simulink model "Control_test"  (R2014b)
settings: Solver=FixedStepDiscrete  StartTime=0.0  StopTime=Inf  FixedStep=0.001  RelTol=1e-3
PostLoadFcn:
  | , if any(exist('dsrtsu_mdlpostloadfcn', 'file') == [2, 3, 6]), try dsrtsu_mdlpostloadfcn('Execute', bdroot); catch fprintf('Error in PostLoadFcn (dsrtsu_mdlpostloadfcn) for model "%s":\n %s\n', bdroot, lasterr); end, end,
undefined symbols (not defined in the file or in its folder): dtLocal, slcm
libraries: rtican x163, simulink x14
(part 15 of 34)

== system Control_test/InputProcessing/RadarCanProcessing/ESR_Status5 ==
  Bus Creator : BusCreator  Inputs=8
  ESR_Status5 : rtican/RTICAN Receive (RX)   Reserved1=[]  Reserved2=[]  Reserved3=[]  Reserved4=[]  SfcnMessage=[]  Msg_Struct=[]  BoardTypeNo=[]  BoardNo=[]  ChannelNo=[]  Parameters=[]  DialogFcn=[]  UnitName=[]  Revision=[]  UnitValues=[]  DSProperties=struct('RTI',struct('Version',uint32(5),'BlockType',struct('isSLSource',uint8(1),'isSLSink',uint8(1),'isHWSource',uint8(0),'isHWSink',uint8(0),'isSetup',uint8(0),'isInline',uint8(1),'isNonInline',uint8(0),'isInterrupt',uint8(0),'isChannelwise',uint8(0)),'IOBoardType','RTICAN','UnitType','MESSAGE','Identifier','RX','DialogType','MSVC','BlockSet','RTICAN','SlaveProcessor','CAN'))  RTIBlockInterface=struct('OutputPortsWidth',int32([1 1 1 1 1 1 1 1]),'OutputPortsActive',[1 1 1 1 1 1 1 1],'OutputPortsName',{{'CAN_TX_SUPPLY_10V_A2D','CAN_TX_SUPPLY_3P3V_A2D','CAN_TX_SUPPLY_5VDX_A2D','CAN_TX_SUPPLY_5VA_A2D','CAN_TX_TEMP2_A2D','CAN_TX_TEMP1_A2D','CAN_TX_IGNP_A2D','CAN_TX_SWBATT_A2D'}},'OutputPortsDataType',{{'SS_DOUBLE','SS_DOUBLE','SS_DOUBLE','SS_DOUBLE','SS_DOUBLE','SS_DOUBLE','SS_DOUBLE','SS_DOUBLE'}},'OutputPortsLabel',{{'CAN_TX_SUPPLY_10V_A2D','CAN_TX_SUPPLY_3P3V_A2D','CAN_TX_SUPPLY_5VDX_A2D','CAN_TX_SUPPLY_5VA_A2D','CAN_TX_TEMP2_A2D','CAN_TX_TEMP1_A2D','CAN_TX_IGNP_A2D','CAN_TX_SWBATT_A2D'}},'OutputPortsLabelMode','ON','InputPortsWidth',int32(0),'InputPortsActive',0,'DialogFcn','rtican_message_interface_gui','BlockDisplay',{{'','center'}},'IconTransparency','on','ParameterTunableNames',{{}},'InitLevel',3,'BlockName',struct('Token',{{'ESR_Status5'}}),'SampleTime',{{-1}},'TriggerPort',{{'none'}},'EnablePort',{{'none'}})  RTIBlockParameters=struct('BoardTypeNo',{{1,'OFF',[]}},'BoardNo',{{2,'ON',[1 16]}},'ChannelNo',{{2,'ON',[1 2]}},'Parameters',{{struct('DataFileSupport',struct('DataFileSelectedMaster',1,'DataFileSelectedLocal',1,'DataFileName',['c:\users\mpc\dropbox\hyundai car setup\esr_dv3_64tgt.dbc|'],'DataFileDate',['26-Aug-2014 13:16:21'],'SelectedFile','..\..\dbcfiles\esr_dv3_64tgt.dbc','InterfaceFcn','rtican_dbc_file_parser'),'Options',struct('StatusSelected',0,'TimeSelected',0,'DeltaTimeSelected',0,'BytePortSelected',0,'MessageLengthSelected',0,'TriggerPort',struct('Selected',0,'TriggerType',0),'UserCoding',struct('Selected',0,'InterfaceFile','UserDecodingFile','FcnName','UserDecodeFcn','InportSelected',0,'InportWidth',1,'OutportSelected',0,'OutportWidth',1),'EnablePortSelected',0,'SignalOnPortnameSelected',1,'UseRXService',0),'Message',struct('MsgOnBlocknameSelected',1,'MsgName','ESR_Status5','MsgIdFormat',0,'MsgId',1508,'MsgLength',8,'NumSignals',8,'SampleTime',-1,'Signal',struct('SgnName',{'CAN_TX_SUPPLY_10V_A2D','CAN_TX_SUPPLY_3P3V_A2D','CAN_TX_SUPPLY_5VDX_A2D','CAN_TX_SUPPLY_5VA_A2D','CAN_TX_TEMP2_A2D','CAN_TX_TEMP1_A2D','CAN_TX_IGNP_A2D','CAN_TX_SWBATT_A2D'},'SgnStartBit',{0,8,16,24,32,40,48,56},'SgnLength',{8,8,8,8,8,8,8,8},'ByteLayout',{2,2,2,2,2,2,2,2},'Factor',{1,1,1,1,1,1,1,1},'Offset',{0,0,0,0,0,0,0,0},'SgnComment',{'','','','','','','',''},'SgnUnit',{'','','','','','','',''},'Min',{0,0,0,0,0,0,0,0},'Max',{0,0,0,0,0,0,0,0},'SgnType',{0,0,0,0,0,0,0,0},'SLDataType',{'SS_DOUBLE','SS_DOUBLE','SS_DOUBLE','SS_DOUBLE','SS_DOUBLE','SS_DOUBLE','SS_DOUBLE','SS_DOUBLE'},'DataType',{0,0,0,0,0,0,0,0},'ModeValue',{-1,-1,-1,-1,-1,-1,-1,-1}),'MsgIdNumFormat',0,'MsgComment',{{''}}),'Version',1.2,'general',struct('isFromLib',0)),'OFF',[]}},'GroupId',{{struct('Group',{{'RTICAN'}},'No',4,'Behavior',{{'NAMECHANGE'}},'BlockType',{{'SINK'}},'NameChangeFlag',0),'OFF',[]}},'SFcnRTICANMessage',{{struct('MsgType','RX','SFcnPortType','Scalar','MsgName','ESR_Status5','MsgIdFormat','STD','MsgId',1508,'MsgLength',8,'NumSignals',8,'SampleTime',-1,'Signal',struct('SgnName',{'CAN_TX_SUPPLY_10V_A2D','CAN_TX_SUPPLY_3P3V_A2D','CAN_TX_SUPPLY_5VDX_A2D','CAN_TX_SUPPLY_5VA_A2D','CAN_TX_TEMP2_A2D','CAN_TX_TEMP1_A2D','CAN_TX_IGNP_A2D','CAN_TX_SWBATT_A2D'},'SgnStartBit',{0,8,16,24,32,40,48,56},'SgnLength',{8,8,8,8,8,8,8,8},'ByteLayout',{['motorola back.'],['motorola back.'],['motorola back.'],['motorola back.'],['motorola back.'],['motorola back.'],['motorola back.'],['motorola back.']},'Factor',{1,1,1,1,1,1,1,1},'Offset',{0,0,0,0,0,0,0,0},'SgnType',{'standard','standard','standard','standard','standard','standard','standard','standard'},'SLDataType',{'SS_DOUBLE','SS_DOUBLE','SS_DOUBLE','SS_DOUBLE','SS_DOUBLE','SS_DOUBLE','SS_DOUBLE','SS_DOUBLE'},'DataType',{['unsigned int'],['unsigned int'],['unsigned int'],['unsigned int'],['unsigned int'],['unsigned int'],['unsigned int'],['unsigned int']},'ModeValue',{-1,-1,-1,-1,-1,-1,-1,-1}),'StatusSelected','no','TimeSelected','no','DeltaTimeSelected','no','BytePortSelected','no','MessageLengthSelected','no','TriggerPort',struct('Selected','no','TriggerType',0),'UserCoding',struct('Selected','no','InterfaceFile','UserDecodingFile','FcnName','UserDecodeFcn','InportSelected','no','InportWidth',1,'OutportSelected','no','OutportWidth',1),'EnablePortSelected','no','UseRXService','no','BoardType','DS1','BoardNo',2,'ControllerNo',2),'OFF',[]}},'TLCFileName',{{'rtican_rx_message','OFF',[]}})  RTISFcnParameters=struct('SFcnRTICANMessage','struct','TLCFileName','char')  RTIBlockParaDefault=struct('BoardTypeNo',4302,'BoardNo',1,'ChannelNo',1,'Parameters',struct('DataFileSupport',struct('DataFileSelectedMaster',0,'DataFileSelectedLocal',0,'DataFileName','','DataFileDate','','SelectedFile',['<no file selected>']),'Options',struct('StatusSelected',1,'TimeSelected',1,'DeltaTimeSelected',1,'BytePortSelected',0,'MessageLengthSelected',0,'TriggerPort',struct('Selected',0,'TriggerType','rising'),'UserCoding',struct('Selected',0,'InterfaceFile','UserDecodingFile','FcnName','UserDecodeFcn','InportSelected',0,'InportWidth',1,'OutportSelected',0,'OutportWidth',1),'EnablePortSelected',0,'SignalOnPortnameSelected',1,'UseRXService',0),'Message',struct('MsgOnBlocknameSelected',0,'MsgName',['RX Message'],'MsgIdFormat',0,'MsgId',100,'MsgLength',8,'NumSignals',1,'SampleTime',-1,'Signal',struct('SgnName',['RX signal'],'SgnStartBit',0,'SgnLength',8,'SgnType',0,'ModeValue',-1,'DataType',0,'SLDataType','SS_DOUBLE','ByteLayout',0,'Factor',1,'Offset',0,'Min',0,'Max',255,'SgnComment',{{}},'SgnUnit',''),'MsgIdNumFormat',0,'MsgComment',{{''}}),'Version',1.2,'general',struct('isFromLib',1)),'GroupId',struct('Group',{{'RTICAN'}},'No',1,'Behavior',{{'NAMECHANGE'}},'BlockType',{{'SINK'}},'NameChangeFlag',0),'SFcnRTICANMessage',struct('MsgType','RX','MsgName',['RX Message'],'MsgIdFormat','STD','MsgId',100,'MsgLength',8,'NumSignals',1,'SampleTime',-1,'Signal',struct('SgnName',['RX signal'],'SgnStartBit',0,'SgnLength',8,'SgnType','standard','ModeValue',-1,'DataType',['unsigned int'],'ByteLayout',['little endian'],'SLDataType','SS_DOUBLE','Factor',1,'Offset',0),'StatusSelected','yes','TimeSelected','yes','DeltaTimeSelected','yes','BytePortSelected','no','MessageLengthSelected','no','EnablePortSelected','no','UserCoding',struct('Selected','no','InterfaceFile','UserDecodingFile','FcnName','UserDecodeFcn','InportSelected','no','InportWidth',1,'OutportSelected','no','OutportWidth',1),'TriggerPort',struct('Selected','no','TriggerType','rising'),'UseRXService','no','BoardType','DS4302','BoardNo',1,'ControllerNo',1,'SFcnPortType','Scalar'),'TLCFileName','rtican_rx_message')
      settings: AttributesFormatString=Group Id: RTICAN4\n
  ESR_Status5_1 : Outport
  wires:
  Bus Creator/1 -> ESR_Status5_1/1  "ESR_Status5"
  ESR_Status5/1 -> Bus Creator/1  "CAN_TX_SUPPLY_10V_A2D"
  ESR_Status5/2 -> Bus Creator/2  "CAN_TX_SUPPLY_3P3V_A2D"
  ESR_Status5/3 -> Bus Creator/3  "CAN_TX_SUPPLY_5VDX_A2D"
  ESR_Status5/4 -> Bus Creator/4  "CAN_TX_SUPPLY_5VA_A2D"
  ESR_Status5/5 -> Bus Creator/5  "CAN_TX_TEMP2_A2D"
  ESR_Status5/6 -> Bus Creator/6  "CAN_TX_TEMP1_A2D"
  ESR_Status5/7 -> Bus Creator/7  "CAN_TX_IGNP_A2D"
  ESR_Status5/8 -> Bus Creator/8  "CAN_TX_SWBATT_A2D"

== system Control_test/InputProcessing/RadarCanProcessing/ESR_Status6 ==
  Bus Creator : BusCreator  Inputs=13
  ESR_Status6 : rtican/RTICAN Receive (RX)   Reserved1=[]  Reserved2=[]  Reserved3=[]  Reserved4=[]  SfcnMessage=[]  Msg_Struct=[]  BoardTypeNo=[]  BoardNo=[]  ChannelNo=[]  Parameters=[]  DialogFcn=[]  UnitName=[]  Revision=[]  UnitValues=[]  DSProperties=struct('RTI',struct('Version',uint32(5),'BlockType',struct('isSLSource',uint8(1),'isSLSink',uint8(1),'isHWSource',uint8(0),'isHWSink',uint8(0),'isSetup',uint8(0),'isInline',uint8(1),'isNonInline',uint8(0),'isInterrupt',uint8(0),'isChannelwise',uint8(0)),'IOBoardType','RTICAN','UnitType','MESSAGE','Identifier','RX','DialogType','MSVC','BlockSet','RTICAN','SlaveProcessor','CAN'))  RTIBlockInterface=struct('OutputPortsWidth',int32([1 1 1 1 1 1 1 1 1 1 1 1 1]),'OutputPortsActive',[1 1 1 1 1 1 1 1 1 1 1 1 1],'OutputPortsName',{{'CAN_TX_VERTICAL_MISALIGNMENT','CAN_TX_SERV_ALIGN_UPDATES_DONE','CAN_TX_FACTORY_MISALIGNMENT','CAN_TX_FACTORY_ALIGN_STATUS_2','CAN_TX_FACTORY_ALIGN_STATUS_1','CAN_TX_RECOMMEND_UNCONVERGE','CAN_TX_FOUND_TARGET','CAN_TX_SYSTEM_POWER_MODE','CAN_TX_VERTICAL_ALIGN_UPDATED','CAN_TX_SW_VERSION_DSP_3RD_BYTE','CAN_TX_WAVE_DIFF_A2D','CAN_TX_SUPPLY_N5V_A2D','CAN_TX_SUPPLY_1P8V_A2D'}},'OutputPortsDataType',{{'SS_DOUBLE','SS_DOUBLE','SS_DOUBLE','SS_DOUBLE','SS_DOUBLE','SS_DOUBLE','SS_DOUBLE','SS_DOUBLE','SS_DOUBLE','SS_DOUBLE','SS_DOUBLE','SS_DOUBLE','SS_DOUBLE'}},'OutputPortsLabel',{{'CAN_TX_VERTICAL_MISALIGNMENT','CAN_TX_SERV_ALIGN_UPDATES_DONE','CAN_TX_FACTORY_MISALIGNMENT','CAN_TX_FACTORY_ALIGN_STATUS_2','CAN_TX_FACTORY_ALIGN_STATUS_1','CAN_TX_RECOMMEND_UNCONVERGE','CAN_TX_FOUND_TARGET','CAN_TX_SYSTEM_POWER_MODE','CAN_TX_VERTICAL_ALIGN_UPDATED','CAN_TX_SW_VERSION_DSP_3RD_BYTE','CAN_TX_WAVE_DIFF_A2D','CAN_TX_SUPPLY_N5V_A2D','CAN_TX_SUPPLY_1P8V_A2D'}},'OutputPortsLabelMode','ON','InputPortsWidth',int32(0),'InputPortsActive',0,'DialogFcn','rtican_message_interface_gui','BlockDisplay',{{'','center'}},'IconTransparency','on','ParameterTunableNames',{{}},'InitLevel',3,'BlockName',struct('Token',{{'ESR_Status6'}}),'SampleTime',{{-1}},'TriggerPort',{{'none'}},'EnablePort',{{'none'}})  RTIBlockParameters=struct('BoardTypeNo',{{1,'OFF',[]}},'BoardNo',{{2,'ON',[1 16]}},'ChannelNo',{{2,'ON',[1 2]}},'Parameters',{{struct('DataFileSupport',struct('DataFileSelectedMaster',1,'DataFileSelectedLocal',1,'DataFileName',['c:\users\mpc\dropbox\hyundai car setup\esr_dv3_64tgt.dbc|'],'DataFileDate',['26-Aug-2014 13:16:21'],'SelectedFile','..\..\dbcfiles\esr_dv3_64tgt.dbc','InterfaceFcn','rtican_dbc_file_parser'),'Options',struct('StatusSelected',0,'TimeSelected',0,'DeltaTimeSelected',0,'BytePortSelected',0,'MessageLengthSelected',0,'TriggerPort',struct('Selected',0,'TriggerType',0),'UserCoding',struct('Selected',0,'InterfaceFile','UserDecodingFile','FcnName','UserDecodeFcn','InportSelected',0,'InportWidth',1,'OutportSelected',0,'OutportWidth',1),'EnablePortSelected',0,'SignalOnPortnameSelected',1,'UseRXService',0),'Message',struct('MsgOnBlocknameSelected',1,'MsgName','ESR_Status6','MsgIdFormat',0,'MsgId',1509,'MsgLength',8,'NumSignals',13,'SampleTime',-1,'Signal',struct('SgnName',{'CAN_TX_VERTICAL_MISALIGNMENT','CAN_TX_SERV_ALIGN_UPDATES_DONE','CAN_TX_FACTORY_MISALIGNMENT','CAN_TX_FACTORY_ALIGN_STATUS_2','CAN_TX_FACTORY_ALIGN_STATUS_1','CAN_TX_RECOMMEND_UNCONVERGE','CAN_TX_FOUND_TARGET','CAN_TX_SYSTEM_POWER_MODE','CAN_TX_VERTICAL_ALIGN_UPDATED','CAN_TX_SW_VERSION_DSP_3RD_BYTE','CAN_TX_WAVE_DIFF_A2D','CAN_TX_SUPPLY_N5V_A2D','CAN_TX_SUPPLY_1P8V_A2D'},'SgnStartBit',{0,8,16,24,27,30,31,32,35,36,40,48,56},'SgnLength',{8,8,8,3,3,1,1,3,1,4,8,8,8},'ByteLayout',{2,2,2,2,2,2,2,2,2,2,2,2,2},'Factor',{0.0625,1,0.0625,1,1,1,1,1,1,1,1,1,1},'Offset',{0,0,0,0,0,0,0,0,0,0,0,0,0},'SgnComment',{'','','','','','','','','','','','',''},'SgnUnit',{'','','deg','','','','','','','','','',''},'Min',{-6,0,-5,0,0,0,0,0,0,0,0,0,0},'Max',{6,255,5,5,5,0,0,0,0,0,0,0,0},'SgnType',{0,0,0,0,0,0,0,0,0,0,0,0,0},'SLDataType',{'SS_DOUBLE','SS_DOUBLE','SS_DOUBLE','SS_DOUBLE','SS_DOUBLE','SS_DOUBLE','SS_DOUBLE','SS_DOUBLE','SS_DOUBLE','SS_DOUBLE','SS_DOUBLE','SS_DOUBLE','SS_DOUBLE'},'DataType',{1,0,1,0,0,0,0,0,0,0,0,0,0},'ModeValue',{-1,-1,-1,-1,-1,-1,-1,-1,-1,-1,-1,-1,-1}),'MsgIdNumFormat',0,'MsgComment',{{''}}),'Version',1.2,'general',struct('isFromLib',0)),'OFF',[]}},'GroupId',{{struct('Group',{{'RTICAN'}},'No',4,'Behavior',{{'NAMECHANGE'}},'BlockType',{{'SINK'}},'NameChangeFlag',0),'OFF',[]}},'SFcnRTICANMessage',{{struct('MsgType','RX','SFcnPortType','Scalar','MsgName','ESR_Status6','MsgIdFormat','STD','MsgId',1509,'MsgLength',8,'NumSignals',13,'SampleTime',-1,'Signal',struct('SgnName',{'CAN_TX_VERTICAL_MISALIGNMENT','CAN_TX_SERV_ALIGN_UPDATES_DONE','CAN_TX_FACTORY_MISALIGNMENT','CAN_TX_FACTORY_ALIGN_STATUS_2','CAN_TX_FACTORY_ALIGN_STATUS_1','CAN_TX_RECOMMEND_UNCONVERGE','CAN_TX_FOUND_TARGET','CAN_TX_SYSTEM_POWER_MODE','CAN_TX_VERTICAL_ALIGN_UPDATED','CAN_TX_SW_VERSION_DSP_3RD_BYTE','CAN_TX_WAVE_DIFF_A2D','CAN_TX_SUPPLY_N5V_A2D','CAN_TX_SUPPLY_1P8V_A2D'},'SgnStartBit',{0,8,16,24,27,30,31,32,35,36,40,48,56},'SgnLength',{8,8,8,3,3,1,1,3,1,4,8,8,8},'ByteLayout',{['motorola back.'],['motorola back.'],['motorola back.'],['motorola back.'],['motorola back.'],['motorola back.'],['motorola back.'],['motorola back.'],['motorola back.'],['motorola back.'],['motorola back.'],['motorola back.'],['motorola back.']},'Factor',{0.0625,1,0.0625,1,1,1,1,1,1,1,1,1,1},'Offset',{0,0,0,0,0,0,0,0,0,0,0,0,0},'SgnType',{'standard','standard','standard','standard','standard','standard','standard','standard','standard','standard','standard','standard','standard'},'SLDataType',{'SS_DOUBLE','SS_DOUBLE','SS_DOUBLE','SS_DOUBLE','SS_DOUBLE','SS_DOUBLE','SS_DOUBLE','SS_DOUBLE','SS_DOUBLE','SS_DOUBLE','SS_DOUBLE','SS_DOUBLE','SS_DOUBLE'},'DataType',{['signed int'],['unsigned int'],['signed int'],['unsigned int'],['unsigned int'],['unsigned int'],['unsigned int'],['unsigned int'],['unsigned int'],['unsigned int'],['unsigned int'],['unsigned int'],['unsigned int']},'ModeValue',{-1,-1,-1,-1,-1,-1,-1,-1,-1,-1,-1,-1,-1}),'StatusSelected','no','TimeSelected','no','DeltaTimeSelected','no','BytePortSelected','no','MessageLengthSelected','no','TriggerPort',struct('Selected','no','TriggerType',0),'UserCoding',struct('Selected','no','InterfaceFile','UserDecodingFile','FcnName','UserDecodeFcn','InportSelected','no','InportWidth',1,'OutportSelected','no','OutportWidth',1),'EnablePortSelected','no','UseRXService','no','BoardType','DS1','BoardNo',2,'ControllerNo',2),'OFF',[]}},'TLCFileName',{{'rtican_rx_message','OFF',[]}})  RTISFcnParameters=struct('SFcnRTICANMessage','struct','TLCFileName','char')  RTIBlockParaDefault=struct('BoardTypeNo',4302,'BoardNo',1,'ChannelNo',1,'Parameters',struct('DataFileSupport',struct('DataFileSelectedMaster',0,'DataFileSelectedLocal',0,'DataFileName','','DataFileDate','','SelectedFile',['<no file selected>']),'Options',struct('StatusSelected',1,'TimeSelected',1,'DeltaTimeSelected',1,'BytePortSelected',0,'MessageLengthSelected',0,'TriggerPort',struct('Selected',0,'TriggerType','rising'),'UserCoding',struct('Selected',0,'InterfaceFile','UserDecodingFile','FcnName','UserDecodeFcn','InportSelected',0,'InportWidth',1,'OutportSelected',0,'OutportWidth',1),'EnablePortSelected',0,'SignalOnPortnameSelected',1,'UseRXService',0),'Message',struct('MsgOnBlocknameSelected',0,'MsgName',['RX Message'],'MsgIdFormat',0,'MsgId',100,'MsgLength',8,'NumSignals',1,'SampleTime',-1,'Signal',struct('SgnName',['RX signal'],'SgnStartBit',0,'SgnLength',8,'SgnType',0,'ModeValue',-1,'DataType',0,'SLDataType','SS_DOUBLE','ByteLayout',0,'Factor',1,'Offset',0,'Min',0,'Max',255,'SgnComment',{{}},'SgnUnit',''),'MsgIdNumFormat',0,'MsgComment',{{''}}),'Version',1.2,'general',struct('isFromLib',1)),'GroupId',struct('Group',{{'RTICAN'}},'No',1,'Behavior',{{'NAMECHANGE'}},'BlockType',{{'SINK'}},'NameChangeFlag',0),'SFcnRTICANMessage',struct('MsgType','RX','MsgName',['RX Message'],'MsgIdFormat','STD','MsgId',100,'MsgLength',8,'NumSignals',1,'SampleTime',-1,'Signal',struct('SgnName',['RX signal'],'SgnStartBit',0,'SgnLength',8,'SgnType','standard','ModeValue',-1,'DataType',['unsigned int'],'ByteLayout',['little endian'],'SLDataType','SS_DOUBLE','Factor',1,'Offset',0),'StatusSelected','yes','TimeSelected','yes','DeltaTimeSelected','yes','BytePortSelected','no','MessageLengthSelected','no','EnablePortSelected','no','UserCoding',struct('Selected','no','InterfaceFile','UserDecodingFile','FcnName','UserDecodeFcn','InportSelected','no','InportWidth',1,'OutportSelected','no','OutportWidth',1),'TriggerPort',struct('Selected','no','TriggerType','rising'),'UseRXService','no','BoardType','DS4302','BoardNo',1,'ControllerNo',1,'SFcnPortType','Scalar'),'TLCFileName','rtican_rx_message')
      settings: AttributesFormatString=Group Id: RTICAN4\n
  ESR_Status6_1 : Outport
  wires:
  Bus Creator/1 -> ESR_Status6_1/1  "ESR_Status6"
  ESR_Status6/1 -> Bus Creator/1  "CAN_TX_VERTICAL_MISALIGNMENT"
  ESR_Status6/2 -> Bus Creator/2  "CAN_TX_SERV_ALIGN_UPDATES_DONE"
  ESR_Status6/3 -> Bus Creator/3  "CAN_TX_FACTORY_MISALIGNMENT"
  ESR_Status6/4 -> Bus Creator/4  "CAN_TX_FACTORY_ALIGN_STATUS_2"
  ESR_Status6/5 -> Bus Creator/5  "CAN_TX_FACTORY_ALIGN_STATUS_1"
  ESR_Status6/6 -> Bus Creator/6  "CAN_TX_RECOMMEND_UNCONVERGE"
  ESR_Status6/7 -> Bus Creator/7  "CAN_TX_FOUND_TARGET"
  ESR_Status6/8 -> Bus Creator/8  "CAN_TX_SYSTEM_POWER_MODE"
  ESR_Status6/9 -> Bus Creator/9  "CAN_TX_VERTICAL_ALIGN_UPDATED"
  ESR_Status6/10 -> Bus Creator/10  "CAN_TX_SW_VERSION_DSP_3RD_BYTE"
  ESR_Status6/11 -> Bus Creator/11  "CAN_TX_WAVE_DIFF_A2D"
  ESR_Status6/12 -> Bus Creator/12  "CAN_TX_SUPPLY_N5V_A2D"
  ESR_Status6/13 -> Bus Creator/13  "CAN_TX_SUPPLY_1P8V_A2D"

== system Control_test/InputProcessing/RadarCanProcessing/ESR_Status7 ==
  Bus Creator : BusCreator  Inputs=8
  ESR_Status7 : rtican/RTICAN Receive (RX)   Reserved1=[]  Reserved2=[]  Reserved3=[]  Reserved4=[]  SfcnMessage=[]  Msg_Struct=[]  BoardTypeNo=[]  BoardNo=[]  ChannelNo=[]  Parameters=[]  DialogFcn=[]  UnitName=[]  Revision=[]  UnitValues=[]  DSProperties=struct('RTI',struct('Version',uint32(5),'BlockType',struct('isSLSource',uint8(1),'isSLSink',uint8(1),'isHWSource',uint8(0),'isHWSink',uint8(0),'isSetup',uint8(0),'isInline',uint8(1),'isNonInline',uint8(0),'isInterrupt',uint8(0),'isChannelwise',uint8(0)),'IOBoardType','RTICAN','UnitType','MESSAGE','Identifier','RX','DialogType','MSVC','BlockSet','RTICAN','SlaveProcessor','CAN'))  RTIBlockInterface=struct('OutputPortsWidth',int32([1 1 1 1 1 1 1 1]),'OutputPortsActive',[1 1 1 1 1 1 1 1],'OutputPortsName',{{'CAN_TX_ACTIVE_FAULT_7','CAN_TX_ACTIVE_FAULT_6','CAN_TX_ACTIVE_FAULT_5','CAN_TX_ACTIVE_FAULT_4','CAN_TX_ACTIVE_FAULT_3','CAN_TX_ACTIVE_FAULT_2','CAN_TX_ACTIVE_FAULT_1','CAN_TX_ACTIVE_FAULT_0'}},'OutputPortsDataType',{{'SS_DOUBLE','SS_DOUBLE','SS_DOUBLE','SS_DOUBLE','SS_DOUBLE','SS_DOUBLE','SS_DOUBLE','SS_DOUBLE'}},'OutputPortsLabel',{{'CAN_TX_ACTIVE_FAULT_7','CAN_TX_ACTIVE_FAULT_6','CAN_TX_ACTIVE_FAULT_5','CAN_TX_ACTIVE_FAULT_4','CAN_TX_ACTIVE_FAULT_3','CAN_TX_ACTIVE_FAULT_2','CAN_TX_ACTIVE_FAULT_1','CAN_TX_ACTIVE_FAULT_0'}},'OutputPortsLabelMode','ON','InputPortsWidth',int32(0),'InputPortsActive',0,'DialogFcn','rtican_message_interface_gui','BlockDisplay',{{'','center'}},'IconTransparency','on','ParameterTunableNames',{{}},'InitLevel',3,'BlockName',struct('Token',{{'ESR_Status7'}}),'SampleTime',{{-1}},'TriggerPort',{{'none'}},'EnablePort',{{'none'}})  RTIBlockParameters=struct('BoardTypeNo',{{1,'OFF',[]}},'BoardNo',{{2,'ON',[1 16]}},'ChannelNo',{{2,'ON',[1 2]}},'Parameters',{{struct('DataFileSupport',struct('DataFileSelectedMaster',1,'DataFileSelectedLocal',1,'DataFileName',['c:\users\mpc\dropbox\hyundai car setup\esr_dv3_64tgt.dbc|'],'DataFileDate',['26-Aug-2014 13:16:21'],'SelectedFile','..\..\dbcfiles\esr_dv3_64tgt.dbc','InterfaceFcn','rtican_dbc_file_parser'),'Options',struct('StatusSelected',0,'TimeSelected',0,'DeltaTimeSelected',0,'BytePortSelected',0,'MessageLengthSelected',0,'TriggerPort',struct('Selected',0,'TriggerType',0),'UserCoding',struct('Selected',0,'InterfaceFile','UserDecodingFile','FcnName','UserDecodeFcn','InportSelected',0,'InportWidth',1,'OutportSelected',0,'OutportWidth',1),'EnablePortSelected',0,'SignalOnPortnameSelected',1,'UseRXService',0),'Message',struct('MsgOnBlocknameSelected',1,'MsgName','ESR_Status7','MsgIdFormat',0,'MsgId',1510,'MsgLength',8,'NumSignals',8,'SampleTime',-1,'Signal',struct('SgnName',{'CAN_TX_ACTIVE_FAULT_7','CAN_TX_ACTIVE_FAULT_6','CAN_TX_ACTIVE_FAULT_5','CAN_TX_ACTIVE_FAULT_4','CAN_TX_ACTIVE_FAULT_3','CAN_TX_ACTIVE_FAULT_2','CAN_TX_ACTIVE_FAULT_1','CAN_TX_ACTIVE_FAULT_0'},'SgnStartBit',{0,8,16,24,32,40,48,56},'SgnLength',{8,8,8,8,8,8,8,8},'ByteLayout',{2,2,2,2,2,2,2,2},'Factor',{1,1,1,1,1,1,1,1},'Offset',{0,0,0,0,0,0,0,0},'SgnComment',{'','','','','','','',''},'SgnUnit',{'','','','','','','',''},'Min',{0,0,0,0,0,0,0,0},'Max',{0,0,0,0,0,0,0,0},'SgnType',{0,0,0,0,0,0,0,0},'SLDataType',{'SS_DOUBLE','SS_DOUBLE','SS_DOUBLE','SS_DOUBLE','SS_DOUBLE','SS_DOUBLE','SS_DOUBLE','SS_DOUBLE'},'DataType',{0,0,0,0,0,0,0,0},'ModeValue',{-1,-1,-1,-1,-1,-1,-1,-1}),'MsgIdNumFormat',0,'MsgComment',{{''}}),'Version',1.2,'general',struct('isFromLib',0)),'OFF',[]}},'GroupId',{{struct('Group',{{'RTICAN'}},'No',4,'Behavior',{{'NAMECHANGE'}},'BlockType',{{'SINK'}},'NameChangeFlag',0),'OFF',[]}},'SFcnRTICANMessage',{{struct('MsgType','RX','SFcnPortType','Scalar','MsgName','ESR_Status7','MsgIdFormat','STD','MsgId',1510,'MsgLength',8,'NumSignals',8,'SampleTime',-1,'Signal',struct('SgnName',{'CAN_TX_ACTIVE_FAULT_7','CAN_TX_ACTIVE_FAULT_6','CAN_TX_ACTIVE_FAULT_5','CAN_TX_ACTIVE_FAULT_4','CAN_TX_ACTIVE_FAULT_3','CAN_TX_ACTIVE_FAULT_2','CAN_TX_ACTIVE_FAULT_1','CAN_TX_ACTIVE_FAULT_0'},'SgnStartBit',{0,8,16,24,32,40,48,56},'SgnLength',{8,8,8,8,8,8,8,8},'ByteLayout',{['motorola back.'],['motorola back.'],['motorola back.'],['motorola back.'],['motorola back.'],['motorola back.'],['motorola back.'],['motorola back.']},'Factor',{1,1,1,1,1,1,1,1},'Offset',{0,0,0,0,0,0,0,0},'SgnType',{'standard','standard','standard','standard','standard','standard','standard','standard'},'SLDataType',{'SS_DOUBLE','SS_DOUBLE','SS_DOUBLE','SS_DOUBLE','SS_DOUBLE','SS_DOUBLE','SS_DOUBLE','SS_DOUBLE'},'DataType',{['unsigned int'],['unsigned int'],['unsigned int'],['unsigned int'],['unsigned int'],['unsigned int'],['unsigned int'],['unsigned int']},'ModeValue',{-1,-1,-1,-1,-1,-1,-1,-1}),'StatusSelected','no','TimeSelected','no','DeltaTimeSelected','no','BytePortSelected','no','MessageLengthSelected','no','TriggerPort',struct('Selected','no','TriggerType',0),'UserCoding',struct('Selected','no','InterfaceFile','UserDecodingFile','FcnName','UserDecodeFcn','InportSelected','no','InportWidth',1,'OutportSelected','no','OutportWidth',1),'EnablePortSelected','no','UseRXService','no','BoardType','DS1','BoardNo',2,'ControllerNo',2),'OFF',[]}},'TLCFileName',{{'rtican_rx_message','OFF',[]}})  RTISFcnParameters=struct('SFcnRTICANMessage','struct','TLCFileName','char')  RTIBlockParaDefault=struct('BoardTypeNo',4302,'BoardNo',1,'ChannelNo',1,'Parameters',struct('DataFileSupport',struct('DataFileSelectedMaster',0,'DataFileSelectedLocal',0,'DataFileName','','DataFileDate','','SelectedFile',['<no file selected>']),'Options',struct('StatusSelected',1,'TimeSelected',1,'DeltaTimeSelected',1,'BytePortSelected',0,'MessageLengthSelected',0,'TriggerPort',struct('Selected',0,'TriggerType','rising'),'UserCoding',struct('Selected',0,'InterfaceFile','UserDecodingFile','FcnName','UserDecodeFcn','InportSelected',0,'InportWidth',1,'OutportSelected',0,'OutportWidth',1),'EnablePortSelected',0,'SignalOnPortnameSelected',1,'UseRXService',0),'Message',struct('MsgOnBlocknameSelected',0,'MsgName',['RX Message'],'MsgIdFormat',0,'MsgId',100,'MsgLength',8,'NumSignals',1,'SampleTime',-1,'Signal',struct('SgnName',['RX signal'],'SgnStartBit',0,'SgnLength',8,'SgnType',0,'ModeValue',-1,'DataType',0,'SLDataType','SS_DOUBLE','ByteLayout',0,'Factor',1,'Offset',0,'Min',0,'Max',255,'SgnComment',{{}},'SgnUnit',''),'MsgIdNumFormat',0,'MsgComment',{{''}}),'Version',1.2,'general',struct('isFromLib',1)),'GroupId',struct('Group',{{'RTICAN'}},'No',1,'Behavior',{{'NAMECHANGE'}},'BlockType',{{'SINK'}},'NameChangeFlag',0),'SFcnRTICANMessage',struct('MsgType','RX','MsgName',['RX Message'],'MsgIdFormat','STD','MsgId',100,'MsgLength',8,'NumSignals',1,'SampleTime',-1,'Signal',struct('SgnName',['RX signal'],'SgnStartBit',0,'SgnLength',8,'SgnType','standard','ModeValue',-1,'DataType',['unsigned int'],'ByteLayout',['little endian'],'SLDataType','SS_DOUBLE','Factor',1,'Offset',0),'StatusSelected','yes','TimeSelected','yes','DeltaTimeSelected','yes','BytePortSelected','no','MessageLengthSelected','no','EnablePortSelected','no','UserCoding',struct('Selected','no','InterfaceFile','UserDecodingFile','FcnName','UserDecodeFcn','InportSelected','no','InportWidth',1,'OutportSelected','no','OutportWidth',1),'TriggerPort',struct('Selected','no','TriggerType','rising'),'UseRXService','no','BoardType','DS4302','BoardNo',1,'ControllerNo',1,'SFcnPortType','Scalar'),'TLCFileName','rtican_rx_message')
      settings: AttributesFormatString=Group Id: RTICAN4\n
  ESR_Status7_1 : Outport
  wires:
  Bus Creator/1 -> ESR_Status7_1/1  "ESR_Status7"
  ESR_Status7/1 -> Bus Creator/1  "CAN_TX_ACTIVE_FAULT_7"
  ESR_Status7/2 -> Bus Creator/2  "CAN_TX_ACTIVE_FAULT_6"
  ESR_Status7/3 -> Bus Creator/3  "CAN_TX_ACTIVE_FAULT_5"
  ESR_Status7/4 -> Bus Creator/4  "CAN_TX_ACTIVE_FAULT_4"
  ESR_Status7/5 -> Bus Creator/5  "CAN_TX_ACTIVE_FAULT_3"
  ESR_Status7/6 -> Bus Creator/6  "CAN_TX_ACTIVE_FAULT_2"
  ESR_Status7/7 -> Bus Creator/7  "CAN_TX_ACTIVE_FAULT_1"
  ESR_Status7/8 -> Bus Creator/8  "CAN_TX_ACTIVE_FAULT_0"

== system Control_test/InputProcessing/RadarCanProcessing/ESR_Status8 ==
  Bus Creator : BusCreator  Inputs=8
  ESR_Status8 : rtican/RTICAN Receive (RX)   Reserved1=[]  Reserved2=[]  Reserved3=[]  Reserved4=[]  SfcnMessage=[]  Msg_Struct=[]  BoardTypeNo=[]  BoardNo=[]  ChannelNo=[]  Parameters=[]  DialogFcn=[]  UnitName=[]  Revision=[]  UnitValues=[]  DSProperties=struct('RTI',struct('Version',uint32(5),'BlockType',struct('isSLSource',uint8(1),'isSLSink',uint8(1),'isHWSource',uint8(0),'isHWSink',uint8(0),'isSetup',uint8(0),'isInline',uint8(1),'isNonInline',uint8(0),'isInterrupt',uint8(0),'isChannelwise',uint8(0)),'IOBoardType','RTICAN','UnitType','MESSAGE','Identifier','RX','DialogType','MSVC','BlockSet','RTICAN','SlaveProcessor','CAN'))  RTIBlockInterface=struct('OutputPortsWidth',int32([1 1 1 1 1 1 1 1]),'OutputPortsActive',[1 1 1 1 1 1 1 1],'OutputPortsName',{{'CAN_TX_HISTORY_FAULT_7','CAN_TX_HISTORY_FAULT_6','CAN_TX_HISTORY_FAULT_5','CAN_TX_HISTORY_FAULT_4','CAN_TX_HISTORY_FAULT_3','CAN_TX_HISTORY_FAULT_2','CAN_TX_HISTORY_FAULT_1','CAN_TX_HISTORY_FAULT_0'}},'OutputPortsDataType',{{'SS_DOUBLE','SS_DOUBLE','SS_DOUBLE','SS_DOUBLE','SS_DOUBLE','SS_DOUBLE','SS_DOUBLE','SS_DOUBLE'}},'OutputPortsLabel',{{'CAN_TX_HISTORY_FAULT_7','CAN_TX_HISTORY_FAULT_6','CAN_TX_HISTORY_FAULT_5','CAN_TX_HISTORY_FAULT_4','CAN_TX_HISTORY_FAULT_3','CAN_TX_HISTORY_FAULT_2','CAN_TX_HISTORY_FAULT_1','CAN_TX_HISTORY_FAULT_0'}},'OutputPortsLabelMode','ON','InputPortsWidth',int32(0),'InputPortsActive',0,'DialogFcn','rtican_message_interface_gui','BlockDisplay',{{'','center'}},'IconTransparency','on','ParameterTunableNames',{{}},'InitLevel',3,'BlockName',struct('Token',{{'ESR_Status8'}}),'SampleTime',{{-1}},'TriggerPort',{{'none'}},'EnablePort',{{'none'}})  RTIBlockParameters=struct('BoardTypeNo',{{1,'OFF',[]}},'BoardNo',{{2,'ON',[1 16]}},'ChannelNo',{{2,'ON',[1 2]}},'Parameters',{{struct('DataFileSupport',struct('DataFileSelectedMaster',1,'DataFileSelectedLocal',1,'DataFileName',['c:\users\mpc\dropbox\hyundai car setup\esr_dv3_64tgt.dbc|'],'DataFileDate',['26-Aug-2014 13:16:21'],'SelectedFile','..\..\dbcfiles\esr_dv3_64tgt.dbc','InterfaceFcn','rtican_dbc_file_parser'),'Options',struct('StatusSelected',0,'TimeSelected',0,'DeltaTimeSelected',0,'BytePortSelected',0,'MessageLengthSelected',0,'TriggerPort',struct('Selected',0,'TriggerType',0),'UserCoding',struct('Selected',0,'InterfaceFile','UserDecodingFile','FcnName','UserDecodeFcn','InportSelected',0,'InportWidth',1,'OutportSelected',0,'OutportWidth',1),'EnablePortSelected',0,'SignalOnPortnameSelected',1,'UseRXService',0),'Message',struct('MsgOnBlocknameSelected',1,'MsgName','ESR_Status8','MsgIdFormat',0,'MsgId',1511,'MsgLength',8,'NumSignals',8,'SampleTime',-1,'Signal',struct('SgnName',{'CAN_TX_HISTORY_FAULT_7','CAN_TX_HISTORY_FAULT_6','CAN_TX_HISTORY_FAULT_5','CAN_TX_HISTORY_FAULT_4','CAN_TX_HISTORY_FAULT_3','CAN_TX_HISTORY_FAULT_2','CAN_TX_HISTORY_FAULT_1','CAN_TX_HISTORY_FAULT_0'},'SgnStartBit',{0,8,16,24,32,40,48,56},'SgnLength',{8,8,8,8,8,8,8,8},'ByteLayout',{2,2,2,2,2,2,2,2},'Factor',{1,1,1,1,1,1,1,1},'Offset',{0,0,0,0,0,0,0,0},'SgnComment',{'','','','','','','',''},'SgnUnit',{'','','','','','','',''},'Min',{0,0,0,0,0,0,0,0},'Max',{0,0,0,0,0,0,0,0},'SgnType',{0,0,0,0,0,0,0,0},'SLDataType',{'SS_DOUBLE','SS_DOUBLE','SS_DOUBLE','SS_DOUBLE','SS_DOUBLE','SS_DOUBLE','SS_DOUBLE','SS_DOUBLE'},'DataType',{0,0,0,0,0,0,0,0},'ModeValue',{-1,-1,-1,-1,-1,-1,-1,-1}),'MsgIdNumFormat',0,'MsgComment',{{''}}),'Version',1.2,'general',struct('isFromLib',0)),'OFF',[]}},'GroupId',{{struct('Group',{{'RTICAN'}},'No',4,'Behavior',{{'NAMECHANGE'}},'BlockType',{{'SINK'}},'NameChangeFlag',0),'OFF',[]}},'SFcnRTICANMessage',{{struct('MsgType','RX','SFcnPortType','Scalar','MsgName','ESR_Status8','MsgIdFormat','STD','MsgId',1511,'MsgLength',8,'NumSignals',8,'SampleTime',-1,'Signal',struct('SgnName',{'CAN_TX_HISTORY_FAULT_7','CAN_TX_HISTORY_FAULT_6','CAN_TX_HISTORY_FAULT_5','CAN_TX_HISTORY_FAULT_4','CAN_TX_HISTORY_FAULT_3','CAN_TX_HISTORY_FAULT_2','CAN_TX_HISTORY_FAULT_1','CAN_TX_HISTORY_FAULT_0'},'SgnStartBit',{0,8,16,24,32,40,48,56},'SgnLength',{8,8,8,8,8,8,8,8},'ByteLayout',{['motorola back.'],['motorola back.'],['motorola back.'],['motorola back.'],['motorola back.'],['motorola back.'],['motorola back.'],['motorola back.']},'Factor',{1,1,1,1,1,1,1,1},'Offset',{0,0,0,0,0,0,0,0},'SgnType',{'standard','standard','standard','standard','standard','standard','standard','standard'},'SLDataType',{'SS_DOUBLE','SS_DOUBLE','SS_DOUBLE','SS_DOUBLE','SS_DOUBLE','SS_DOUBLE','SS_DOUBLE','SS_DOUBLE'},'DataType',{['unsigned int'],['unsigned int'],['unsigned int'],['unsigned int'],['unsigned int'],['unsigned int'],['unsigned int'],['unsigned int']},'ModeValue',{-1,-1,-1,-1,-1,-1,-1,-1}),'StatusSelected','no','TimeSelected','no','DeltaTimeSelected','no','BytePortSelected','no','MessageLengthSelected','no','TriggerPort',struct('Selected','no','TriggerType',0),'UserCoding',struct('Selected','no','InterfaceFile','UserDecodingFile','FcnName','UserDecodeFcn','InportSelected','no','InportWidth',1,'OutportSelected','no','OutportWidth',1),'EnablePortSelected','no','UseRXService','no','BoardType','DS1','BoardNo',2,'ControllerNo',2),'OFF',[]}},'TLCFileName',{{'rtican_rx_message','OFF',[]}})  RTISFcnParameters=struct('SFcnRTICANMessage','struct','TLCFileName','char')  RTIBlockParaDefault=struct('BoardTypeNo',4302,'BoardNo',1,'ChannelNo',1,'Parameters',struct('DataFileSupport',struct('DataFileSelectedMaster',0,'DataFileSelectedLocal',0,'DataFileName','','DataFileDate','','SelectedFile',['<no file selected>']),'Options',struct('StatusSelected',1,'TimeSelected',1,'DeltaTimeSelected',1,'BytePortSelected',0,'MessageLengthSelected',0,'TriggerPort',struct('Selected',0,'TriggerType','rising'),'UserCoding',struct('Selected',0,'InterfaceFile','UserDecodingFile','FcnName','UserDecodeFcn','InportSelected',0,'InportWidth',1,'OutportSelected',0,'OutportWidth',1),'EnablePortSelected',0,'SignalOnPortnameSelected',1,'UseRXService',0),'Message',struct('MsgOnBlocknameSelected',0,'MsgName',['RX Message'],'MsgIdFormat',0,'MsgId',100,'MsgLength',8,'NumSignals',1,'SampleTime',-1,'Signal',struct('SgnName',['RX signal'],'SgnStartBit',0,'SgnLength',8,'SgnType',0,'ModeValue',-1,'DataType',0,'SLDataType','SS_DOUBLE','ByteLayout',0,'Factor',1,'Offset',0,'Min',0,'Max',255,'SgnComment',{{}},'SgnUnit',''),'MsgIdNumFormat',0,'MsgComment',{{''}}),'Version',1.2,'general',struct('isFromLib',1)),'GroupId',struct('Group',{{'RTICAN'}},'No',1,'Behavior',{{'NAMECHANGE'}},'BlockType',{{'SINK'}},'NameChangeFlag',0),'SFcnRTICANMessage',struct('MsgType','RX','MsgName',['RX Message'],'MsgIdFormat','STD','MsgId',100,'MsgLength',8,'NumSignals',1,'SampleTime',-1,'Signal',struct('SgnName',['RX signal'],'SgnStartBit',0,'SgnLength',8,'SgnType','standard','ModeValue',-1,'DataType',['unsigned int'],'ByteLayout',['little endian'],'SLDataType','SS_DOUBLE','Factor',1,'Offset',0),'StatusSelected','yes','TimeSelected','yes','DeltaTimeSelected','yes','BytePortSelected','no','MessageLengthSelected','no','EnablePortSelected','no','UserCoding',struct('Selected','no','InterfaceFile','UserDecodingFile','FcnName','UserDecodeFcn','InportSelected','no','InportWidth',1,'OutportSelected','no','OutportWidth',1),'TriggerPort',struct('Selected','no','TriggerType','rising'),'UseRXService','no','BoardType','DS4302','BoardNo',1,'ControllerNo',1,'SFcnPortType','Scalar'),'TLCFileName','rtican_rx_message')
      settings: AttributesFormatString=Group Id: RTICAN4\n
  ESR_Status8_1 : Outport
  wires:
  Bus Creator/1 -> ESR_Status8_1/1  "ESR_Status8"
  ESR_Status8/1 -> Bus Creator/1  "CAN_TX_HISTORY_FAULT_7"
  ESR_Status8/2 -> Bus Creator/2  "CAN_TX_HISTORY_FAULT_6"
  ESR_Status8/3 -> Bus Creator/3  "CAN_TX_HISTORY_FAULT_5"
  ESR_Status8/4 -> Bus Creator/4  "CAN_TX_HISTORY_FAULT_4"
  ESR_Status8/5 -> Bus Creator/5  "CAN_TX_HISTORY_FAULT_3"
  ESR_Status8/6 -> Bus Creator/6  "CAN_TX_HISTORY_FAULT_2"
  ESR_Status8/7 -> Bus Creator/7  "CAN_TX_HISTORY_FAULT_1"
  ESR_Status8/8 -> Bus Creator/8  "CAN_TX_HISTORY_FAULT_0"

== system Control_test/InputProcessing/RadarCanProcessing/ESR_Status9 ==
  Bus Creator : BusCreator  Inputs=7
  ESR_Status9 : rtican/RTICAN Receive (RX)   Reserved1=[]  Reserved2=[]  Reserved3=[]  Reserved4=[]  SfcnMessage=[]  Msg_Struct=[]  BoardTypeNo=[]  BoardNo=[]  ChannelNo=[]  Parameters=[]  DialogFcn=[]  UnitName=[]  Revision=[]  UnitValues=[]  DSProperties=struct('RTI',struct('Version',uint32(5),'BlockType',struct('isSLSource',uint8(1),'isSLSink',uint8(1),'isHWSource',uint8(0),'isHWSink',uint8(0),'isSetup',uint8(0),'isInline',uint8(1),'isNonInline',uint8(0),'isInterrupt',uint8(0),'isChannelwise',uint8(0)),'IOBoardType','RTICAN','UnitType','MESSAGE','Identifier','RX','DialogType','MSVC','BlockSet','RTICAN','SlaveProcessor','CAN'))  RTIBlockInterface=struct('OutputPortsWidth',int32([1 1 1 1 1 1 1]),'OutputPortsActive',[1 1 1 1 1 1 1],'OutputPortsName',{{'CAN_TX_PATH_ID_ACC_3','CAN_TX_PATH_ID_ACC_2','CAN_TX_FILTERED_XOHP_ACC_CIPV','CAN_TX_WATER_SPRAY_TARGET_ID','CAN_TX_SERIAL_NUM_3RD_BYTE','CAN_TX_SIDESLIP_ANGLE','CAN_TX_AVG_PWR_CWBLKG'}},'OutputPortsDataType',{{'SS_DOUBLE','SS_DOUBLE','SS_DOUBLE','SS_DOUBLE','SS_DOUBLE','SS_DOUBLE','SS_DOUBLE'}},'OutputPortsLabel',{{'CAN_TX_PATH_ID_ACC_3','CAN_TX_PATH_ID_ACC_2','CAN_TX_FILTERED_XOHP_ACC_CIPV','CAN_TX_WATER_SPRAY_TARGET_ID','CAN_TX_SERIAL_NUM_3RD_BYTE','CAN_TX_SIDESLIP_ANGLE','CAN_TX_AVG_PWR_CWBLKG'}},'OutputPortsLabelMode','ON','InputPortsWidth',int32(0),'InputPortsActive',0,'DialogFcn','rtican_message_interface_gui','BlockDisplay',{{'','center'}},'IconTransparency','on','ParameterTunableNames',{{}},'InitLevel',3,'BlockName',struct('Token',{{'ESR_Status9'}}),'SampleTime',{{-1}},'TriggerPort',{{'none'}},'EnablePort',{{'none'}})  RTIBlockParameters=struct('BoardTypeNo',{{1,'OFF',[]}},'BoardNo',{{2,'ON',[1 16]}},'ChannelNo',{{2,'ON',[1 2]}},'Parameters',{{struct('DataFileSupport',struct('DataFileSelectedMaster',1,'DataFileSelectedLocal',1,'DataFileName',['c:\users\mpc\dropbox\hyundai car setup\esr_dv3_64tgt.dbc|'],'DataFileDate',['26-Aug-2014 13:16:21'],'SelectedFile','..\..\dbcfiles\esr_dv3_64tgt.dbc','InterfaceFcn','rtican_dbc_file_parser'),'Options',struct('StatusSelected',0,'TimeSelected',0,'DeltaTimeSelected',0,'BytePortSelected',0,'MessageLengthSelected',0,'TriggerPort',struct('Selected',0,'TriggerType',0),'UserCoding',struct('Selected',0,'InterfaceFile','UserDecodingFile','FcnName','UserDecodeFcn','InportSelected',0,'InportWidth',1,'OutportSelected',0,'OutportWidth',1),'EnablePortSelected',0,'SignalOnPortnameSelected',1,'UseRXService',0),'Message',struct('MsgOnBlocknameSelected',1,'MsgName','ESR_Status9','MsgIdFormat',0,'MsgId',1512,'MsgLength',8,'NumSignals',7,'SampleTime',-1,'Signal',struct('SgnName',{'CAN_TX_PATH_ID_ACC_3','CAN_TX_PATH_ID_ACC_2','CAN_TX_FILTERED_XOHP_ACC_CIPV','CAN_TX_WATER_SPRAY_TARGET_ID','CAN_TX_SERIAL_NUM_3RD_BYTE','CAN_TX_SIDESLIP_ANGLE','CAN_TX_AVG_PWR_CWBLKG'},'SgnStartBit',{0,8,16,25,32,40,52},'SgnLength',{8,8,9,7,8,10,12},'ByteLayout',{2,2,2,2,2,2,2},'Factor',{1,1,0.03125,1,1,0.125,1},'Offset',{0,0,0,0,0,0,0},'SgnComment',{'','','','','','',''},'SgnUnit',{'','','m','','','deg',''},'Min',{0,0,-8,0,0,-64,0},'Max',{64,64,7.96875,64,0,63.875,0},'SgnType',{0,0,0,0,0,0,0},'SLDataType',{'SS_DOUBLE','SS_DOUBLE','SS_DOUBLE','SS_DOUBLE','SS_DOUBLE','SS_DOUBLE','SS_DOUBLE'},'DataType',{0,0,1,0,0,1,0},'ModeValue',{-1,-1,-1,-1,-1,-1,-1}),'MsgIdNumFormat',0,'MsgComment',{{''}}),'Version',1.2,'general',struct('isFromLib',0)),'OFF',[]}},'GroupId',{{struct('Group',{{'RTICAN'}},'No',4,'Behavior',{{'NAMECHANGE'}},'BlockType',{{'SINK'}},'NameChangeFlag',0),'OFF',[]}},'SFcnRTICANMessage',{{struct('MsgType','RX','SFcnPortType','Scalar','MsgName','ESR_Status9','MsgIdFormat','STD','MsgId',1512,'MsgLength',8,'NumSignals',7,'SampleTime',-1,'Signal',struct('SgnName',{'CAN_TX_PATH_ID_ACC_3','CAN_TX_PATH_ID_ACC_2','CAN_TX_FILTERED_XOHP_ACC_CIPV','CAN_TX_WATER_SPRAY_TARGET_ID','CAN_TX_SERIAL_NUM_3RD_BYTE','CAN_TX_SIDESLIP_ANGLE','CAN_TX_AVG_PWR_CWBLKG'},'SgnStartBit',{0,8,16,25,32,40,52},'SgnLength',{8,8,9,7,8,10,12},'ByteLayout',{['motorola back.'],['motorola back.'],['motorola back.'],['motorola back.'],['motorola back.'],['motorola back.'],['motorola back.']},'Factor',{1,1,0.03125,1,1,0.125,1},'Offset',{0,0,0,0,0,0,0},'SgnType',{'standard','standard','standard','standard','standard','standard','standard'},'SLDataType',{'SS_DOUBLE','SS_DOUBLE','SS_DOUBLE','SS_DOUBLE','SS_DOUBLE','SS_DOUBLE','SS_DOUBLE'},'DataType',{['unsigned int'],['unsigned int'],['signed int'],['unsigned int'],['unsigned int'],['signed int'],['unsigned int']},'ModeValue',{-1,-1,-1,-1,-1,-1,-1}),'StatusSelected','no','TimeSelected','no','DeltaTimeSelected','no','BytePortSelected','no','MessageLengthSelected','no','TriggerPort',struct('Selected','no','TriggerType',0),'UserCoding',struct('Selected','no','InterfaceFile','UserDecodingFile','FcnName','UserDecodeFcn','InportSelected','no','InportWidth',1,'OutportSelected','no','OutportWidth',1),'EnablePortSelected','no','UseRXService','no','BoardType','DS1','BoardNo',2,'ControllerNo',2),'OFF',[]}},'TLCFileName',{{'rtican_rx_message','OFF',[]}})  RTISFcnParameters=struct('SFcnRTICANMessage','struct','TLCFileName','char')  RTIBlockParaDefault=struct('BoardTypeNo',4302,'BoardNo',1,'ChannelNo',1,'Parameters',struct('DataFileSupport',struct('DataFileSelectedMaster',0,'DataFileSelectedLocal',0,'DataFileName','','DataFileDate','','SelectedFile',['<no file selected>']),'Options',struct('StatusSelected',1,'TimeSelected',1,'DeltaTimeSelected',1,'BytePortSelected',0,'MessageLengthSelected',0,'TriggerPort',struct('Selected',0,'TriggerType','rising'),'UserCoding',struct('Selected',0,'InterfaceFile','UserDecodingFile','FcnName','UserDecodeFcn','InportSelected',0,'InportWidth',1,'OutportSelected',0,'OutportWidth',1),'EnablePortSelected',0,'SignalOnPortnameSelected',1,'UseRXService',0),'Message',struct('MsgOnBlocknameSelected',0,'MsgName',['RX Message'],'MsgIdFormat',0,'MsgId',100,'MsgLength',8,'NumSignals',1,'SampleTime',-1,'Signal',struct('SgnName',['RX signal'],'SgnStartBit',0,'SgnLength',8,'SgnType',0,'ModeValue',-1,'DataType',0,'SLDataType','SS_DOUBLE','ByteLayout',0,'Factor',1,'Offset',0,'Min',0,'Max',255,'SgnComment',{{}},'SgnUnit',''),'MsgIdNumFormat',0,'MsgComment',{{''}}),'Version',1.2,'general',struct('isFromLib',1)),'GroupId',struct('Group',{{'RTICAN'}},'No',1,'Behavior',{{'NAMECHANGE'}},'BlockType',{{'SINK'}},'NameChangeFlag',0),'SFcnRTICANMessage',struct('MsgType','RX','MsgName',['RX Message'],'MsgIdFormat','STD','MsgId',100,'MsgLength',8,'NumSignals',1,'SampleTime',-1,'Signal',struct('SgnName',['RX signal'],'SgnStartBit',0,'SgnLength',8,'SgnType','standard','ModeValue',-1,'DataType',['unsigned int'],'ByteLayout',['little endian'],'SLDataType','SS_DOUBLE','Factor',1,'Offset',0),'StatusSelected','yes','TimeSelected','yes','DeltaTimeSelected','yes','BytePortSelected','no','MessageLengthSelected','no','EnablePortSelected','no','UserCoding',struct('Selected','no','InterfaceFile','UserDecodingFile','FcnName','UserDecodeFcn','InportSelected','no','InportWidth',1,'OutportSelected','no','OutportWidth',1),'TriggerPort',struct('Selected','no','TriggerType','rising'),'UseRXService','no','BoardType','DS4302','BoardNo',1,'ControllerNo',1,'SFcnPortType','Scalar'),'TLCFileName','rtican_rx_message')
      settings: AttributesFormatString=Group Id: RTICAN4\n
  ESR_Status9_1 : Outport
  wires:
  Bus Creator/1 -> ESR_Status9_1/1  "ESR_Status9"
  ESR_Status9/1 -> Bus Creator/1  "CAN_TX_PATH_ID_ACC_3"
  ESR_Status9/2 -> Bus Creator/2  "CAN_TX_PATH_ID_ACC_2"
  ESR_Status9/3 -> Bus Creator/3  "CAN_TX_FILTERED_XOHP_ACC_CIPV"
  ESR_Status9/4 -> Bus Creator/4  "CAN_TX_WATER_SPRAY_TARGET_ID"
  ESR_Status9/5 -> Bus Creator/5  "CAN_TX_SERIAL_NUM_3RD_BYTE"
  ESR_Status9/6 -> Bus Creator/6  "CAN_TX_SIDESLIP_ANGLE"
  ESR_Status9/7 -> Bus Creator/7  "CAN_TX_AVG_PWR_CWBLKG"
